simulink model "PID_sin_boques"  (Simulink 7.8)
settings: Solver=ode45  StartTime=0.0  StopTime=10  RelTol=1e-3
values from neighbouring files (symbols this model uses):
  b = 1.2*10^(-4)    (= 0.00012)    [Initial_datab.m]
  d = 3*10^(-6)    (= 3e-06)    [Initial_datab.m]
  Ixx = 10.4*10^(-3)    (= 0.0104)    [Initial_datab.m]
  Iyy = 11.2*10^(-3)    (= 0.0112)    [Initial_datab.m]
  Izz = 2.29*10^(-2)    (= 0.0229)    [Initial_datab.m]
  Jr = 7.25*10^(-5)    (= 7.25e-05)    [Initial_datab.m]
  Kp_phi = 4    [Const_PID.m]
  Kp_psi = 1.5    [Const_PID.m]
  Kp_theta = 2    [Const_PID.m]
  Kp_z = 8    [Const_PID.m]
  l = 0.225    [Initial_datab.m]
  m = 1.14    [Initial_datab.m]
  phi0 = 0    [Initial_datab.m]
  phi0dot = 0    [Initial_datab.m]
  psi0 = 0    [Initial_datab.m]
  psi0dot = 0    [Initial_datab.m]
  Td_phi = 0.1833    [Const_PID.m]
  Td_psi = 0.42    [Const_PID.m]
  Td_theta = 0.275    [Const_PID.m]
  Td_z = 0.5    [Const_PID.m]
  theta0 = 0    [Initial_datab.m]
  theta0dot = 0    [Initial_datab.m]
  Ti_phi = 100000000    [Const_PID.m]
  Ti_psi = 1000000    [Const_PID.m]
  Ti_theta = 10000000    [Const_PID.m]
  Ti_z = 1000000000    [Const_PID.m]
  x0 = 0    [Initial_datab.m]
  x0dot = 0    [Initial_datab.m]
  y0 = 0    [Initial_datab.m]
  y0dot = 0    [Initial_datab.m]
  z0 = 0    [Initial_datab.m]
  z0dot = 0    [Initial_datab.m]
undefined symbols (not defined in the file or in its folder): sigbuilder_block
libraries: aerolibconvert2 x9, simulink x1
settings Model: Creator=Ana  LastModifiedBy=Ana

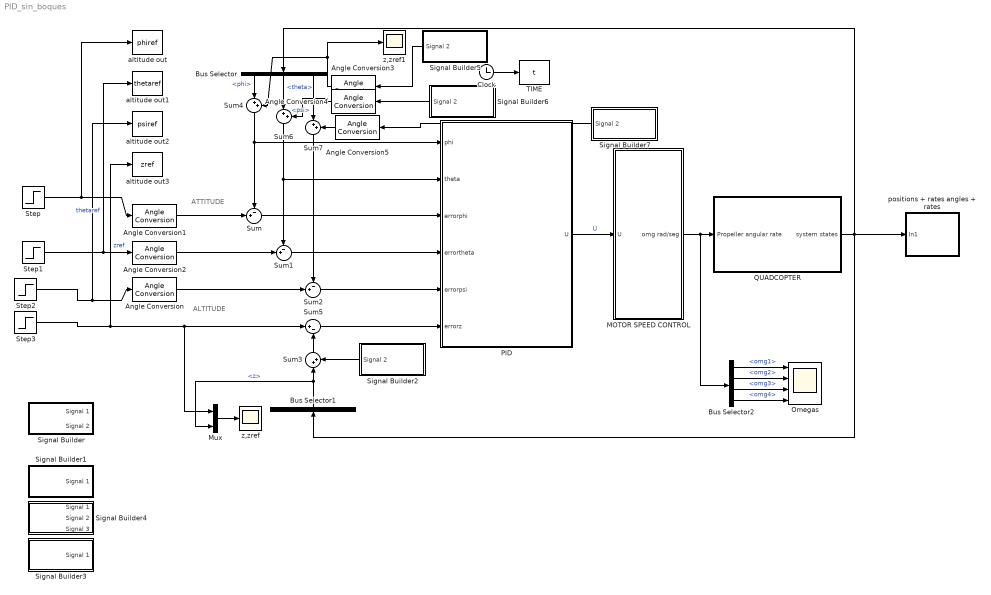
== system PID_sin_boques ==
  note: ATTITUDE
  note: ALTITUDE
  Angle Conversion{,1..5} (6 alike) : aerolibconvert2/Angle Conversion  IU=deg  OU=rad
  Bus Selector : BusSelector  OutputSignals=States.phi,States.theta,States.psi
  Bus Selector1 : BusSelector  OutputSignals=States.z
  Bus Selector2 : BusSelector  OutputSignals=omg1,omg2,omg3,omg4
  Clock : Clock
  MOTOR SPEED CONTROL : Subsystem
  Mux : Mux  Inputs=2
  Omegas : Scope  NumInputPorts=4
      settings: YMin=-5~-5~-5~-5  YMax=5~5~5~5  SaveName=ScopeData17
  PID : Subsystem
  QUADCOPTER : Subsystem
  Signal Builder : Subsystem  Tag=STV Subsys  LoadFcn=sigbuilder_block('load');  StartFcn=sigbuilder_block('start');  StopFcn=sigbuilder_block('stop');  ClipboardFcn=sigbuilder_block('clipboard');  mask(Sigbuilder block){}
      mask help: Simulink:masks:SigbuilderBlock_MD
      mask init:
      | if ~strcmp(get_param(bdroot(gcbh),'SimulationStatus'),'stopped') tuvar = sigbuilder_block('maskInit'); end
      settings: CopyFcn=sigbuilder_block('copy');  DeleteFcn=sigbuilder_block('delete');  ModelCloseFcn=sigbuilder_block('modelClose');  PreSaveFcn=sigbuilder_block('preSave');  NameChangeFcn=sigbuilder_block('namechange');  OpenFcn=sigbuilder_block('open',[437.25 117.75 550.5 394.5 ]);  CloseFcn=sigbuilder_block('close');
      mask Display: plot(0, 0, 100, 100,[2, 2, 32, 32, 2], [68, 8, 8, 68, 68],[32, 2], [38, 38], [32, 19, 2],[53, 60, 44], [32, 17, 17, 2],[16, 16, 31, 31]);txt = getActiveGroup(gcbh);text(2, 100, txt,'verticalAlignment', 'top');
  Signal Builder1 : Subsystem  Tag=STV Subsys  LoadFcn=sigbuilder_block('load');  StartFcn=sigbuilder_block('start');  StopFcn=sigbuilder_block('stop');  ClipboardFcn=sigbuilder_block('clipboard');  mask(Sigbuilder block){}
      mask help: Simulink:masks:SigbuilderBlock_MD
      mask init:
      | if ~strcmp(get_param(bdroot(gcbh),'SimulationStatus'),'stopped') tuvar = sigbuilder_block('maskInit'); end
      settings: CopyFcn=sigbuilder_block('copy');  DeleteFcn=sigbuilder_block('delete');  ModelCloseFcn=sigbuilder_block('modelClose');  PreSaveFcn=sigbuilder_block('preSave');  NameChangeFcn=sigbuilder_block('namechange');  OpenFcn=sigbuilder_block('open',[437.25 117.75 550.5 394.5 ]);  CloseFcn=sigbuilder_block('close');
      mask Display: plot(0, 0, 100, 100,[2, 2, 32, 32, 2], [68, 8, 8, 68, 68],[32, 2], [38, 38], [32, 19, 2],[53, 60, 44], [32, 17, 17, 2],[16, 16, 31, 31]);txt = getActiveGroup(gcbh);text(2, 100, txt,'verticalAlignment', 'top');
  Signal Builder2 : Subsystem  Tag=STV Subsys  LoadFcn=sigbuilder_block('load');  StartFcn=sigbuilder_block('start');  StopFcn=sigbuilder_block('stop');  ClipboardFcn=sigbuilder_block('clipboard');  mask(Sigbuilder block){}
      mask help: Simulink:masks:SigbuilderBlock_MD
      mask init:
      | if ~strcmp(get_param(bdroot(gcbh),'SimulationStatus'),'stopped') tuvar = sigbuilder_block('maskInit'); end
      settings: CopyFcn=sigbuilder_block('copy');  DeleteFcn=sigbuilder_block('delete');  ModelCloseFcn=sigbuilder_block('modelClose');  PreSaveFcn=sigbuilder_block('preSave');  NameChangeFcn=sigbuilder_block('namechange');  OpenFcn=sigbuilder_block('open',[437.25 117.75 550.5 394.5 ]);  CloseFcn=sigbuilder_block('close');
      mask Display: plot(0, 0, 100, 100,[2, 2, 32, 32, 2], [68, 8, 8, 68, 68],[32, 2], [38, 38], [32, 19, 2],[53, 60, 44], [32, 17, 17, 2],[16, 16, 31, 31]);txt = getActiveGroup(gcbh);text(2, 100, txt,'verticalAlignment', 'top');
  Signal Builder3 : Subsystem  Tag=STV Subsys  LoadFcn=sigbuilder_block('load');  StartFcn=sigbuilder_block('start');  StopFcn=sigbuilder_block('stop');  ClipboardFcn=sigbuilder_block('clipboard');  mask(Sigbuilder block){}
      mask help: Simulink:masks:SigbuilderBlock_MD
      mask init:
      | if ~strcmp(get_param(bdroot(gcbh),'SimulationStatus'),'stopped') tuvar = sigbuilder_block('maskInit'); end
      settings: CopyFcn=sigbuilder_block('copy');  DeleteFcn=sigbuilder_block('delete');  ModelCloseFcn=sigbuilder_block('modelClose');  PreSaveFcn=sigbuilder_block('preSave');  NameChangeFcn=sigbuilder_block('namechange');  OpenFcn=sigbuilder_block('open',[437.25 117.75 550.5 394.5 ]);  CloseFcn=sigbuilder_block('close');
      mask Display: plot(0, 0, 100, 100,[2, 2, 32, 32, 2], [68, 8, 8, 68, 68],[32, 2], [38, 38], [32, 19, 2],[53, 60, 44], [32, 17, 17, 2],[16, 16, 31, 31]);txt = getActiveGroup(gcbh);text(2, 100, txt,'verticalAlignment', 'top');
  Signal Builder4 : Subsystem  Tag=STV Subsys  LoadFcn=sigbuilder_block('load');  StartFcn=sigbuilder_block('start');  StopFcn=sigbuilder_block('stop');  ClipboardFcn=sigbuilder_block('clipboard');  mask(Sigbuilder block){}
      mask help: Simulink:masks:SigbuilderBlock_MD
      mask init:
      | if ~strcmp(get_param(bdroot(gcbh),'SimulationStatus'),'stopped') tuvar = sigbuilder_block('maskInit'); end
      settings: CopyFcn=sigbuilder_block('copy');  DeleteFcn=sigbuilder_block('delete');  ModelCloseFcn=sigbuilder_block('modelClose');  PreSaveFcn=sigbuilder_block('preSave');  NameChangeFcn=sigbuilder_block('namechange');  OpenFcn=sigbuilder_block('open',[437.25 117.75 550.5 394.5 ]);  CloseFcn=sigbuilder_block('close');
      mask Display: plot(0, 0, 100, 100,[2, 2, 32, 32, 2], [68, 8, 8, 68, 68],[32, 2], [38, 38], [32, 19, 2],[53, 60, 44], [32, 17, 17, 2],[16, 16, 31, 31]);txt = getActiveGroup(gcbh);text(2, 100, txt,'verticalAlignment', 'top');
  Signal Builder5 : Subsystem  Tag=STV Subsys  LoadFcn=sigbuilder_block('load');  StartFcn=sigbuilder_block('start');  StopFcn=sigbuilder_block('stop');  ClipboardFcn=sigbuilder_block('clipboard');  mask(Sigbuilder block){}
      mask help: Simulink:masks:SigbuilderBlock_MD
      mask init:
      | if ~strcmp(get_param(bdroot(gcbh),'SimulationStatus'),'stopped') tuvar = sigbuilder_block('maskInit'); end
      settings: CopyFcn=sigbuilder_block('copy');  DeleteFcn=sigbuilder_block('delete');  ModelCloseFcn=sigbuilder_block('modelClose');  PreSaveFcn=sigbuilder_block('preSave');  NameChangeFcn=sigbuilder_block('namechange');  OpenFcn=sigbuilder_block('open',[437.25 117.75 550.5 394.5 ]);  CloseFcn=sigbuilder_block('close');
      mask Display: plot(0, 0, 100, 100,[2, 2, 32, 32, 2], [68, 8, 8, 68, 68],[32, 2], [38, 38], [32, 19, 2],[53, 60, 44], [32, 17, 17, 2],[16, 16, 31, 31]);txt = getActiveGroup(gcbh);text(2, 100, txt,'verticalAlignment', 'top');
  Signal Builder6 : Subsystem  Tag=STV Subsys  LoadFcn=sigbuilder_block('load');  StartFcn=sigbuilder_block('start');  StopFcn=sigbuilder_block('stop');  ClipboardFcn=sigbuilder_block('clipboard');  mask(Sigbuilder block){}
      mask help: Simulink:masks:SigbuilderBlock_MD
      mask init:
      | if ~strcmp(get_param(bdroot(gcbh),'SimulationStatus'),'stopped') tuvar = sigbuilder_block('maskInit'); end
      settings: CopyFcn=sigbuilder_block('copy');  DeleteFcn=sigbuilder_block('delete');  ModelCloseFcn=sigbuilder_block('modelClose');  PreSaveFcn=sigbuilder_block('preSave');  NameChangeFcn=sigbuilder_block('namechange');  OpenFcn=sigbuilder_block('open',[437.25 117.75 550.5 394.5 ]);  CloseFcn=sigbuilder_block('close');
      mask Display: plot(0, 0, 100, 100,[2, 2, 32, 32, 2], [68, 8, 8, 68, 68],[32, 2], [38, 38], [32, 19, 2],[53, 60, 44], [32, 17, 17, 2],[16, 16, 31, 31]);txt = getActiveGroup(gcbh);text(2, 100, txt,'verticalAlignment', 'top');
  Signal Builder7 : Subsystem  Tag=STV Subsys  LoadFcn=sigbuilder_block('load');  StartFcn=sigbuilder_block('start');  StopFcn=sigbuilder_block('stop');  ClipboardFcn=sigbuilder_block('clipboard');  mask(Sigbuilder block){}
      mask help: Simulink:masks:SigbuilderBlock_MD
      mask init:
      | if ~strcmp(get_param(bdroot(gcbh),'SimulationStatus'),'stopped') tuvar = sigbuilder_block('maskInit'); end
      settings: CopyFcn=sigbuilder_block('copy');  DeleteFcn=sigbuilder_block('delete');  ModelCloseFcn=sigbuilder_block('modelClose');  PreSaveFcn=sigbuilder_block('preSave');  NameChangeFcn=sigbuilder_block('namechange');  OpenFcn=sigbuilder_block('open',[437.25 117.75 550.5 394.5 ]);  CloseFcn=sigbuilder_block('close');
      mask Display: plot(0, 0, 100, 100,[2, 2, 32, 32, 2], [68, 8, 8, 68, 68],[32, 2], [38, 38], [32, 19, 2],[53, 60, 44], [32, 17, 17, 2],[16, 16, 31, 31]);txt = getActiveGroup(gcbh);text(2, 100, txt,'verticalAlignment', 'top');
  Step{,1..3} (4 alike) : Step  SampleTime=0
  Sum : Sum  Inputs=-+|
  Sum1 : Sum  Inputs=-+|
  Sum2 : Sum  Inputs=-+|
  Sum{3..4,6..7} (4 alike) : Sum  Inputs=|++
  Sum5 : Sum  Inputs=|+-
  TIME : ToWorkspace  VariableName=t  SampleTime=-1  SaveFormat=Array
  altitude out : ToWorkspace  VariableName=phiref  SampleTime=-1  SaveFormat=Array
  altitude out1 : ToWorkspace  VariableName=thetaref  SampleTime=-1  SaveFormat=Array
  altitude out2 : ToWorkspace  VariableName=psiref  SampleTime=-1  SaveFormat=Array
  altitude out3 : ToWorkspace  VariableName=zref  SampleTime=-1  SaveFormat=Array
  positions + rates angles + rates : Subsystem
      mask Display: disp('system states')
  z,zref : Scope
      settings: YMin=8.5  YMax=17.5  SaveName=ScopeData3
  z,zref1 : Scope
      settings: YMin=8.5  YMax=17.5  SaveName=ScopeData18
  wires:
  QUADCOPTER/1(system states) -> Bus Selector/1, Bus Selector1/1, positions + rates angles + rates/1(In1)
  Bus Selector/1 -> Sum4/1  "<phi>"
  Step1/1 -> Angle Conversion2/1, altitude out1/1  "thetaref"
  Sum/1 -> PID/3(errorphi)
  Sum1/1 -> PID/4(errortheta)
  Sum2/1 -> PID/5(errorpsi)
  PID/1(U) -> MOTOR SPEED CONTROL/1(U)  "U"
  Step3/1 -> Sum5/1, Mux/1, altitude out3/1  "zref"
  Mux/1 -> z,zref/1
  Sum5/1 -> PID/6(errorz)
  Angle Conversion/1 -> Sum2/2
  Angle Conversion2/1 -> Sum1/2
  Angle Conversion1/1 -> Sum/2
  Bus Selector1/1 -> Sum3/1, Mux/2  "<z>"
  Sum3/1 -> Sum5/2
  Sum4/1 -> Sum/1, PID/1(phi)
  Bus Selector/2 -> Sum6/1  "<theta>"
  Sum6/1 -> Sum1/1, PID/2(theta)
  Bus Selector/3 -> Sum7/1  "<psi>"
  Sum7/1 -> Sum2/1
  Clock/1 -> TIME/1
  MOTOR SPEED CONTROL/1(omg rad/seg) -> QUADCOPTER/1(Propeller angular rate), Bus Selector2/1
  Bus Selector2/1 -> Omegas/1  "<omg1>"
  Bus Selector2/2 -> Omegas/2  "<omg2>"
  Bus Selector2/3 -> Omegas/3  "<omg3>"
  Bus Selector2/4 -> Omegas/4  "<omg4>"
  Step2/1 -> Angle Conversion/1, altitude out2/1
  Step/1 -> Angle Conversion1/1, altitude out/1
  Signal Builder6/1(Signal 2) -> Angle Conversion4/1
  Signal Builder7/1(Signal 2) -> Angle Conversion5/1
  Angle Conversion3/1 -> z,zref1/1, Sum4/2
  Angle Conversion5/1 -> Sum7/2
  Angle Conversion4/1 -> Sum6/2
  Signal Builder2/1(Signal 2) -> Sum3/2
  Signal Builder5/1(Signal 2) -> Angle Conversion3/1

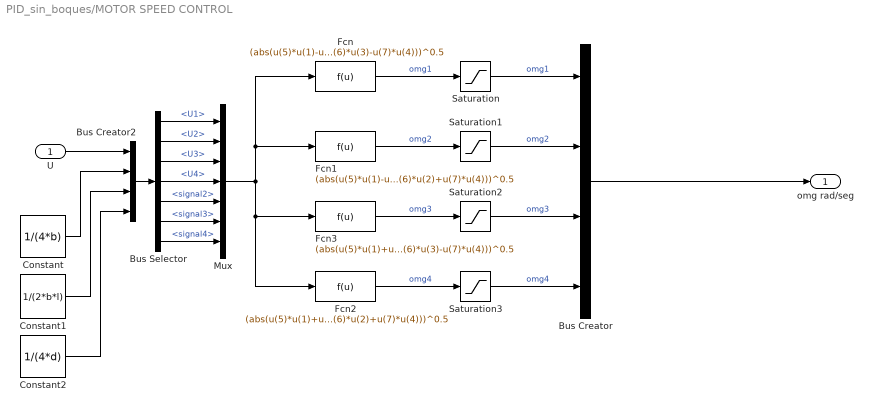
== system PID_sin_boques/MOTOR SPEED CONTROL ==
  U : Inport
  Bus Creator : BusCreator
  Bus Creator2 : BusCreator
  Bus Selector : BusSelector  OutputSignals=U.U1,U.U2,U.U3,U.U4,signal2,signal3,signal4
  Constant : Constant  Value=1/(4*b)
  Constant1 : Constant  Value=1/(2*b*l)
  Constant2 : Constant  Value=1/(4*d)
  Fcn : Fcn  Expr=(abs(u(5)*u(1)-u(6)*u(3)-u(7)*u(4)))^0.5
  Fcn1 : Fcn  Expr=(abs(u(5)*u(1)-u(6)*u(2)+u(7)*u(4)))^0.5
  Fcn2 : Fcn  Expr=(abs(u(5)*u(1)+u(6)*u(2)+u(7)*u(4)))^0.5
  Fcn3 : Fcn  Expr=(abs(u(5)*u(1)+u(6)*u(3)-u(7)*u(4)))^0.5
  Mux : Mux  Inputs=7
  Saturation{,1..3} (4 alike) : Saturate  UpperLimit=215.86  LowerLimit=0  ZeroCross=off
  omg rad/seg : Outport
  wires:
  Constant/1 -> Bus Creator2/2
  Constant1/1 -> Bus Creator2/3
  Bus Creator2/1 -> Bus Selector/1
  Constant2/1 -> Bus Creator2/4
  Bus Selector/1 -> Mux/1  "<U1>"
  Bus Selector/2 -> Mux/2  "<U2>"
  Bus Selector/3 -> Mux/3  "<U3>"
  Bus Selector/4 -> Mux/4  "<U4>"
  Bus Selector/5 -> Mux/5  "<signal2>"
  Bus Selector/6 -> Mux/6  "<signal3>"
  Bus Selector/7 -> Mux/7  "<signal4>"
  U/1 -> Bus Creator2/1
  Bus Creator/1 -> omg rad/seg/1
  Fcn/1 -> Saturation/1  "omg1"
  Fcn1/1 -> Saturation1/1  "omg2"
  Fcn3/1 -> Saturation2/1  "omg3"
  Fcn2/1 -> Saturation3/1  "omg4"
  Saturation/1 -> Bus Creator/1  "omg1"
  Saturation1/1 -> Bus Creator/2  "omg2"
  Saturation2/1 -> Bus Creator/3  "omg3"
  Saturation3/1 -> Bus Creator/4  "omg4"
  Mux/1 -> Fcn1/1, Fcn/1, Fcn3/1, Fcn2/1

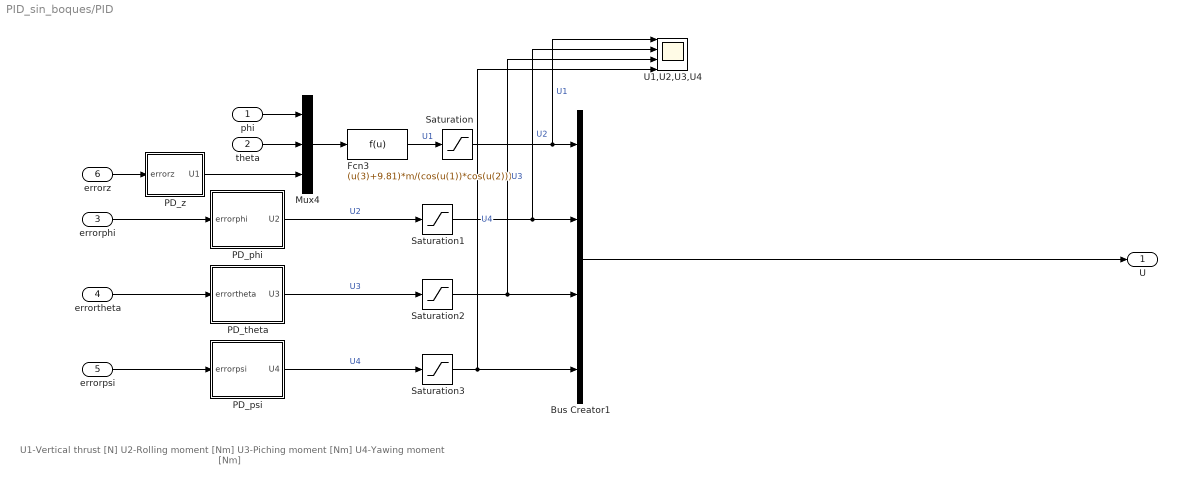
== system PID_sin_boques/PID ==
  note: U1-Vertical thrust [N]
      | U2-Rolling moment [Nm]
      | U3-Piching moment [Nm]
      | U4-Yawing moment [Nm]
  phi : Inport
  theta : Inport  Port=2
  errorphi : Inport  Port=3
  errortheta : Inport  Port=4
  errorpsi : Inport  Port=5
  errorz : Inport  Port=6
  Bus Creator1 : BusCreator
  Fcn3 : Fcn  Expr=(u(3)+9.81)*m/(cos(u(1))*cos(u(2)))
  Mux4 : Mux  Inputs=3
  PD_phi : Subsystem
  PD_psi : Subsystem
  PD_theta : Subsystem
  PD_z : Subsystem
  Saturation : Saturate  UpperLimit=22.36  LowerLimit=0  ZeroCross=off
  Saturation1 : Saturate  UpperLimit=5.5915  LowerLimit=-5.5915  ZeroCross=off
  Saturation2 : Saturate  UpperLimit=5.5915  LowerLimit=-5.5915  ZeroCross=off
  Saturation3 : Saturate  UpperLimit=5.5915  LowerLimit=-5.5915  ZeroCross=off
  U1,U2,U3,U4 : Scope  NumInputPorts=4
      settings: YMin=-5~-5~-5~-5  YMax=5~5~5~5  SaveName=ScopeData22
  U : Outport
  wires:
  Bus Creator1/1 -> U/1
  errorphi/1 -> PD_phi/1(errorphi)
  errortheta/1 -> PD_theta/1(errortheta)
  errorpsi/1 -> PD_psi/1(errorpsi)
  PD_psi/1(U4) -> Saturation3/1  "U4"
  PD_theta/1(U3) -> Saturation2/1  "U3"
  PD_phi/1(U2) -> Saturation1/1  "U2"
  Fcn3/1 -> Saturation/1  "U1"
  Mux4/1 -> Fcn3/1
  errorz/1 -> PD_z/1(errorz)
  PD_z/1(U1) -> Mux4/3
  theta/1 -> Mux4/2
  phi/1 -> Mux4/1
  Saturation/1 -> Bus Creator1/1, U1,U2,U3,U4/1  "U1"
  Saturation1/1 -> Bus Creator1/2, U1,U2,U3,U4/2  "U2"
  Saturation2/1 -> Bus Creator1/3, U1,U2,U3,U4/3  "U3"
  Saturation3/1 -> Bus Creator1/4, U1,U2,U3,U4/4  "U4"

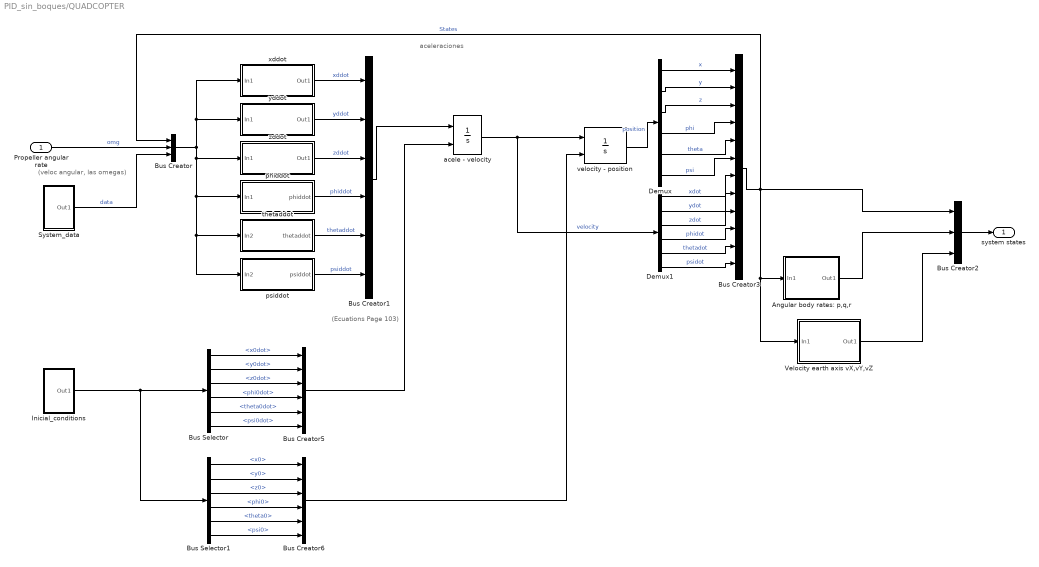
== system PID_sin_boques/QUADCOPTER ==
  note: aceleraciones
  note: (Ecuations Page 103)
  note: (veloc angular, las omegas)
  Propeller angular rate : Inport
  Angular body rates: p,q,r : Subsystem
  Bus Creator : BusCreator  Inputs=3
  Bus Creator1 : BusCreator  Inputs=6
  Bus Creator2 : BusCreator  Inputs=3
  Bus Creator3 : BusCreator  Inputs=12
  Bus Creator5 : BusCreator  Inputs=6
  Bus Creator6 : BusCreator  Inputs=6
  Bus Selector : BusSelector  OutputSignals=x0dot,y0dot,z0dot,phi0dot,theta0dot,psi0dot
  Bus Selector1 : BusSelector  OutputSignals=x0,y0,z0,phi0,theta0,psi0
  Demux : Demux  Outputs=6
  Demux1 : Demux  Outputs=6
  Inicial_conditions : Subsystem
  System_data : Subsystem
  Velocity earth axis vX,vY,vZ : Subsystem
  acele - velocity : Integrator  InitialConditionSource=external
  phiddot : Subsystem
  psiddot : Subsystem
  thetaddot : Subsystem
  velocity - position : Integrator  InitialConditionSource=external
  xddot : Subsystem
  yddot : Subsystem
  zddot : Subsystem
  system states : Outport
  wires:
  Demux/1 -> Bus Creator3/1  "x"
  Demux/2 -> Bus Creator3/2  "y"
  Demux/3 -> Bus Creator3/3  "z"
  Demux1/1 -> Bus Creator3/7  "xdot"
  Demux1/2 -> Bus Creator3/8  "ydot"
  Demux1/3 -> Bus Creator3/9  "zdot"
  Demux1/4 -> Bus Creator3/10  "phidot"
  Demux1/5 -> Bus Creator3/11  "thetadot"
  Demux1/6 -> Bus Creator3/12  "psidot"
  Bus Creator3/1 -> Bus Creator/1, Bus Creator2/1, Angular body rates: p,q,r/1(In1), Velocity earth axis vX,vY,vZ/1(In1)  "States"
  Bus Selector/1 -> Bus Creator5/1  "<x0dot>"
  Bus Selector/2 -> Bus Creator5/2  "<y0dot>"
  Bus Selector/3 -> Bus Creator5/3  "<z0dot>"
  Bus Selector/4 -> Bus Creator5/4  "<phi0dot>"
  Bus Selector/5 -> Bus Creator5/5  "<theta0dot>"
  Bus Selector/6 -> Bus Creator5/6  "<psi0dot>"
  Bus Selector1/1 -> Bus Creator6/1  "<x0>"
  Bus Selector1/2 -> Bus Creator6/2  "<y0>"
  Bus Selector1/3 -> Bus Creator6/3  "<z0>"
  Bus Selector1/4 -> Bus Creator6/4  "<phi0>"
  Bus Selector1/5 -> Bus Creator6/5  "<theta0>"
  Bus Selector1/6 -> Bus Creator6/6  "<psi0>"
  Bus Creator5/1 -> acele - velocity/2
  velocity - position/1 -> Demux/1  "position"
  Bus Creator6/1 -> velocity - position/2
  acele - velocity/1 -> velocity - position/1, Demux1/1  "velocity"
  yddot/1(Out1) -> Bus Creator1/2  "yddot"
  zddot/1(Out1) -> Bus Creator1/3  "zddot"
  phiddot/1(phiddot) -> Bus Creator1/4  "phiddot"
  thetaddot/1(thetaddot) -> Bus Creator1/5  "thetaddot"
  psiddot/1(psiddot) -> Bus Creator1/6  "psiddot"
  Bus Creator1/1 -> acele - velocity/1
  xddot/1(Out1) -> Bus Creator1/1  "xddot"
  Propeller angular rate/1 -> Bus Creator/2  "omg"
  System_data/1(Out1) -> Bus Creator/3  "data"
  Bus Creator/1 -> xddot/1(In1), yddot/1(In1), thetaddot/1(In2), psiddot/1(In2), phiddot/1(In1), zddot/1(In1)
  Angular body rates: p,q,r/1(Out1) -> Bus Creator2/2
  Bus Creator2/1 -> system states/1
  Inicial_conditions/1(Out1) -> Bus Selector/1, Bus Selector1/1
  Velocity earth axis vX,vY,vZ/1(Out1) -> Bus Creator2/3
  Demux/4 -> Bus Creator3/4  "phi"
  Demux/6 -> Bus Creator3/6  "psi"
  Demux/5 -> Bus Creator3/5  "theta"

== system PID_sin_boques/Signal Builder ==
  Demux : Demux  Tag=STV Demux  Outputs=2
  FromWs : FromWorkspace  Tag=STV FromWs  VariableName=tuvar  SampleTime=0  SigBuilderData=DataTag0  VnvData=DataTag1
      SigBuilderData=|
      | common.afterFinalStr = 'Extrapolate'
      | common.sampleTime = 0
      | dataSet.timeRange = [0 10]
      | dataSet.name = 'Group 1'
      | sbobj.Groups.Name = 'Group 1'
      | sbobj.Groups.Signals(1).Name = 'Signal 1'
      | sbobj.Groups.Signals(1).XData = [0 2 4 6 8 10]
      | sbobj.Groups.Signals(1).YData = [0 0 1 1 0 0]
      | sbobj.Groups.Signals(2).Name = 'Signal 2'
      | sbobj.Groups.Signals(2).XData = [0 0.5 1 1.5 2 2.5 3 3.5 4 4.5 5 5.5 6 6.5 7 7.5 8 8.5 9 9.5 10]
      | sbobj.Groups.Signals(2).YData = [0 0.707106781187 1 0.707106781187 1.22464679915e-16 -0.707106781187 -1 -0.707106781187 0 0.707106781187 1 0.707106781187 1.22464679915e-16 -0.707106781187 -1 -0.707106781187 0 0.707106781187 1 0.707106781187 1.22464679915e-16]
  Signal 1 : Outport  Tag=STV Outport
  Signal 2 : Outport  Tag=STV Outport  Port=2
  wires:
  Demux/1 -> Signal 1/1
  FromWs/1 -> Demux/1
  Demux/2 -> Signal 2/1

== system PID_sin_boques/Signal Builder1 ==
  Demux : Demux  Tag=STV Demux  Outputs=1
  FromWs : FromWorkspace  Tag=STV FromWs  VariableName=tuvar  SampleTime=0  SigBuilderData=DataTag2  VnvData=DataTag3
      SigBuilderData=|
      | common.afterFinalStr = 'Extrapolate'
      | common.sampleTime = 0
      | dataSet.timeRange = [0 10]
      | dataSet.name = 'Group 1'
      | sbobj.Groups.Name = 'Group 1'
      | sbobj.Groups.Signals.Name = 'Signal 1'
      | sbobj.Groups.Signals.XData = [0 4 6 6 10]
      | sbobj.Groups.Signals.YData = [0 1 1 0.5 0]
  Signal 1 : Outport  Tag=STV Outport
  wires:
  Demux/1 -> Signal 1/1
  FromWs/1 -> Demux/1

== system PID_sin_boques/Signal Builder2 ==
  Demux : Demux  Tag=STV Demux  Outputs=1
  FromWs : FromWorkspace  Tag=STV FromWs  VariableName=tuvar  SampleTime=0  SigBuilderData=DataTag4  VnvData=DataTag5
      SigBuilderData=|
      | common.afterFinalStr = 'Extrapolate'
      | common.sampleTime = 0
      | dataSet.timeRange = [0 10]
      | dataSet.name = 'Group 1'
      | sbobj.Groups.Name = 'Group 1'
      | sbobj.Groups.Signals.Name = 'Signal 2'
      | sbobj.Groups.Signals.XData = [0 3 3 3.5 3.5 10]
      | sbobj.Groups.Signals.YData = [0 0 1 1 0 0]
  Signal 2 : Outport  Tag=STV Outport
  wires:
  FromWs/1 -> Demux/1
  Demux/1 -> Signal 2/1

== system PID_sin_boques/Signal Builder3 ==
  Demux : Demux  Tag=STV Demux  Outputs=1
  FromWs : FromWorkspace  Tag=STV FromWs  VariableName=tuvar  SampleTime=0  SigBuilderData=DataTag6  VnvData=DataTag7
      SigBuilderData=|
      | common.afterFinalStr = 'Extrapolate'
      | common.sampleTime = 0
      | dataSet.timeRange = [0 10]
      | dataSet.name = 'Group 1'
      | sbobj.Groups.Name = 'Group 1'
      | sbobj.Groups.Signals.Name = 'Signal 1'
      | sbobj.Groups.Signals.XData = [0 3 4 6 8 10]
      | sbobj.Groups.Signals.YData = [0 1 1.98 1.98 0.5 0]
  Signal 1 : Outport  Tag=STV Outport
  wires:
  Demux/1 -> Signal 1/1
  FromWs/1 -> Demux/1

== system PID_sin_boques/Signal Builder4 ==
  Demux : Demux  Tag=STV Demux  Outputs=3
  FromWs : FromWorkspace  Tag=STV FromWs  VariableName=tuvar  SampleTime=0  SigBuilderData=DataTag8  VnvData=DataTag9
      SigBuilderData=|
      | common.afterFinalStr = 'Extrapolate'
      | common.sampleTime = 0
      | dataSet.timeRange = [0 10]
      | dataSet.name = 'Group 1'
      | sbobj.Groups.Name = 'Group 1'
      | sbobj.Groups.Signals(1).Name = 'Signal 1'
      | sbobj.Groups.Signals(1).XData = [0 2 4 6 8 10]
      | sbobj.Groups.Signals(1).YData = [0 0 1 1 0 0]
      | sbobj.Groups.Signals(2).Name = 'Signal 2'
      | sbobj.Groups.Signals(2).XData = [0 4 4 6 6 10]
      | sbobj.Groups.Signals(2).YData = [0 0 1 1 0 0]
      | sbobj.Groups.Signals(3).Name = 'Signal 3'
      | sbobj.Groups.Signals(3).XData = [0 1 2 2 4 4 6 6 8 8 8.56 10]
      | sbobj.Groups.Signals(3).YData = [0 0 0 1 1 0 0 1 1 0 0 0]
  Signal 1 : Outport  Tag=STV Outport
  Signal 2 : Outport  Tag=STV Outport  Port=2
  Signal 3 : Outport  Tag=STV Outport  Port=3
  wires:
  FromWs/1 -> Demux/1
  Demux/1 -> Signal 1/1
  Demux/2 -> Signal 2/1
  Demux/3 -> Signal 3/1

== system PID_sin_boques/Signal Builder5 ==
  Demux : Demux  Tag=STV Demux  Outputs=1
  FromWs : FromWorkspace  Tag=STV FromWs  VariableName=tuvar  SampleTime=0  SigBuilderData=DataTag10  VnvData=DataTag11
      SigBuilderData=|
      | common.afterFinalStr = 'Extrapolate'
      | common.sampleTime = 0
      | dataSet.timeRange = [0 10]
      | dataSet.name = 'Group 1'
      | sbobj.Groups.Name = 'Group 1'
      | sbobj.Groups.Signals.Name = 'Signal 2'
      | sbobj.Groups.Signals.XData = [0 5 5 5.5 5.5 10]
      | sbobj.Groups.Signals.YData = [0 0 3 3 0 0]
  Signal 2 : Outport  Tag=STV Outport
  wires:
  FromWs/1 -> Demux/1
  Demux/1 -> Signal 2/1

== system PID_sin_boques/Signal Builder6 ==
  Demux : Demux  Tag=STV Demux  Outputs=1
  FromWs : FromWorkspace  Tag=STV FromWs  VariableName=tuvar  SampleTime=0  SigBuilderData=DataTag12  VnvData=DataTag13
      SigBuilderData=|
      | common.afterFinalStr = 'Extrapolate'
      | common.sampleTime = 0
      | dataSet.timeRange = [0 10]
      | dataSet.name = 'Group 1'
      | sbobj.Groups.Name = 'Group 1'
      | sbobj.Groups.Signals.Name = 'Signal 2'
      | sbobj.Groups.Signals.XData = [0 7 7 7.5 7.5 10]
      | sbobj.Groups.Signals.YData = [0 0 3 3 0 0]
  Signal 2 : Outport  Tag=STV Outport
  wires:
  FromWs/1 -> Demux/1
  Demux/1 -> Signal 2/1

== system PID_sin_boques/Signal Builder7 ==
  Demux : Demux  Tag=STV Demux  Outputs=1
  FromWs : FromWorkspace  Tag=STV FromWs  VariableName=tuvar  SampleTime=0  SigBuilderData=DataTag14  VnvData=DataTag15
      SigBuilderData=|
      | common.afterFinalStr = 'Extrapolate'
      | common.sampleTime = 0
      | dataSet.timeRange = [0 10]
      | dataSet.name = 'Group 1'
      | sbobj.Groups.Name = 'Group 1'
      | sbobj.Groups.Signals.Name = 'Signal 2'
      | sbobj.Groups.Signals.XData = [0 9 9 9.5 9.5 10]
      | sbobj.Groups.Signals.YData = [0 0 3 3 0 0]
  Signal 2 : Outport  Tag=STV Outport
  wires:
  FromWs/1 -> Demux/1
  Demux/1 -> Signal 2/1

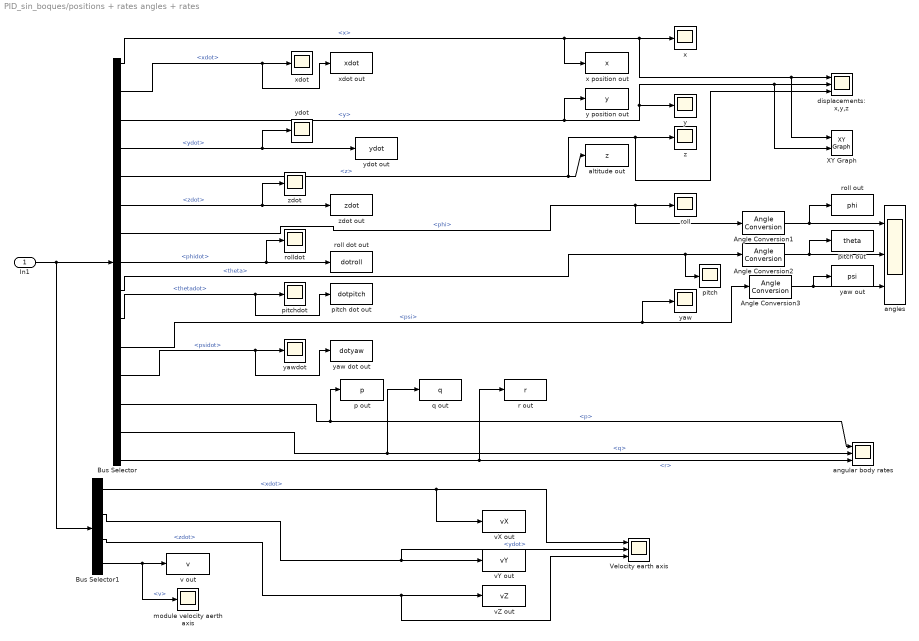
== system PID_sin_boques/positions + rates angles + rates ==
  In1 : Inport
  Angle Conversion1 : aerolibconvert2/Angle Conversion  IU=rad  OU=deg
  Angle Conversion2 : aerolibconvert2/Angle Conversion  IU=rad  OU=deg
  Angle Conversion3 : aerolibconvert2/Angle Conversion  IU=rad  OU=deg
  Bus Selector : BusSelector  OutputSignals=States.x,States.xdot,States.y,States.ydot,States.z,States.zdot,States.phi,States.phidot,States.theta,States.thetadot,States.psi,States.psidot,signal2.p,signal2.q,signal2.r
  Bus Selector1 : BusSelector  OutputSignals=States.xdot,States.ydot,States.zdot,signal3.v
  Velocity earth axis : Scope  NumInputPorts=3
      settings: TimeRange=0.5  YMin=-2.92169e+092~-1.59453e+092~5.72254e+092  YMax=-2.64343e+092~-1.44267e+092~6.32492e+092  SaveName=ScopeData15
  XY Graph : simulink/Sinks/XY Graph  xmin=-8  xmax=8  ymin=-8  ymax=8  st=-1
  altitude out : ToWorkspace  VariableName=z  SampleTime=-1  SaveFormat=Array
  angles : Scope  NumInputPorts=3
      settings: TimeRange=0.1  YMin=0.951985~0.949043~0.952413  YMax=1.05219~1.04894~1.05267  SaveName=ScopeData13
  angular body rates : Scope  NumInputPorts=3
      settings: TimeRange=5  YMin=-5~-0.02~-0.001  YMax=20~0.005000000000000001~0.004  SaveName=ScopeData14
  displacements: x,y,z : Scope  NumInputPorts=3
      settings: TimeRange=0.5  YMin=-1~-1~5.425  YMax=1~1~5.65  SaveName=ScopeData19
  module velocity aerth axis : Scope
      settings: SaveName=ScopeData16
  p out : ToWorkspace  VariableName=p  SampleTime=-1  SaveFormat=Structure
  pitch : Scope
      settings: TimeRange=4  YMin=-0.055  YMax=0.045
  pitch dot out : ToWorkspace  VariableName=dotpitch  SampleTime=-1  SaveFormat=Array
  pitch out : ToWorkspace  VariableName=theta  SampleTime=-1  SaveFormat=Array
  pitchdot : Scope
      settings: YMin=-1.75  YMax=1.75  SaveName=ScopeData4
  q out : ToWorkspace  VariableName=q  SampleTime=-1  SaveFormat=Structure
  r out : ToWorkspace  VariableName=r  SampleTime=-1  SaveFormat=Structure
  roll : Scope
      settings: TimeRange=0.25  YMin=-0.031  YMax=-0.008
  roll dot out : ToWorkspace  VariableName=dotroll  SampleTime=-1  SaveFormat=Array
  roll out : ToWorkspace  VariableName=phi  SampleTime=-1  SaveFormat=Array
  rolldot : Scope
      settings: TimeRange=7  YMin=-0.15  YMax=0.125  SaveName=ScopeData5
  v out : ToWorkspace  VariableName=v  SampleTime=-1  SaveFormat=Array
  vX out : ToWorkspace  VariableName=vX  SampleTime=-1  SaveFormat=Array
  vY out : ToWorkspace  VariableName=vY  SampleTime=-1  SaveFormat=Array
  vZ out : ToWorkspace  VariableName=vZ  SampleTime=-1  SaveFormat=Array
  x : Scope
      settings: TimeRange=20  YMin=-0.5  YMax=2.5  SaveName=ScopeData6
  x position out : ToWorkspace  VariableName=x  SampleTime=-1  SaveFormat=Array
  xdot : Scope
      settings: TimeRange=5  YMin=-4.75e-015  YMax=0  SaveName=ScopeData7
  xdot out : ToWorkspace  VariableName=xdot  SampleTime=-1  SaveFormat=Array
  y : Scope
      settings: TimeRange=5  YMin=1.825  YMax=2.075  SaveName=ScopeData8
  y position out : ToWorkspace  VariableName=y  SampleTime=-1  SaveFormat=Array
  yaw : Scope
      settings: TimeRange=5  YMin=-0.02  YMax=0.0125  SaveName=ScopeData2
  yaw dot out : ToWorkspace  VariableName=dotyaw  SampleTime=-1  SaveFormat=Array
  yaw out : ToWorkspace  VariableName=psi  SampleTime=-1  SaveFormat=Array
  yawdot : Scope
      settings: TimeRange=18  YMin=-0.275  YMax=0.15  SaveName=ScopeData9
  ydot : Scope
      settings: TimeRange=5  YMin=-143.75  YMax=-141.75  SaveName=ScopeData10
  ydot out : ToWorkspace  VariableName=ydot  SampleTime=-1  SaveFormat=Array
  z : Scope
      settings: TimeRange=5  YMin=0.2  YMax=1.5  SaveName=ScopeData11
  zdot : Scope
      settings: TimeRange=10  YMin=-110.5  YMax=-107.25  SaveName=ScopeData12
  zdot out : ToWorkspace  VariableName=zdot  SampleTime=-1  SaveFormat=Array
  wires:
  Bus Selector/3 -> y position out/1, y/1, displacements: x,y,z/2, XY Graph/2  "<y>"
  Bus Selector/12 -> yawdot/1, yaw dot out/1  "<psidot>"
  In1/1 -> Bus Selector/1, Bus Selector1/1
  Bus Selector/10 -> pitchdot/1, pitch dot out/1  "<thetadot>"
  Bus Selector/15 -> angular body rates/3, r out/1  "<r>"
  Bus Selector/14 -> angular body rates/2, q out/1  "<q>"
  Bus Selector/13 -> angular body rates/1, p out/1  "<p>"
  Bus Selector/1 -> x position out/1, x/1, displacements: x,y,z/1, XY Graph/1  "<x>"
  Bus Selector/2 -> xdot out/1, xdot/1  "<xdot>"
  Bus Selector/4 -> ydot out/1, ydot/1  "<ydot>"
  Bus Selector/5 -> altitude out/1, z/1, displacements: x,y,z/3  "<z>"
  Bus Selector/6 -> zdot/1, zdot out/1  "<zdot>"
  Bus Selector/8 -> rolldot/1, roll dot out/1  "<phidot>"
  Bus Selector/9 -> pitch/1, Angle Conversion2/1  "<theta>"
  Bus Selector/11 -> yaw/1, Angle Conversion3/1  "<psi>"
  Bus Selector/7 -> roll/1, Angle Conversion1/1  "<phi>"
  Bus Selector1/2 -> vY out/1, Velocity earth axis/2  "<ydot>"
  Bus Selector1/3 -> vZ out/1, Velocity earth axis/3  "<zdot>"
  Bus Selector1/4 -> v out/1, module velocity aerth axis/1  "<v>"
  Bus Selector1/1 -> vX out/1, Velocity earth axis/1  "<xdot>"
  Angle Conversion1/1 -> angles/1, roll out/1
  Angle Conversion2/1 -> angles/2, pitch out/1
  Angle Conversion3/1 -> angles/3, yaw out/1

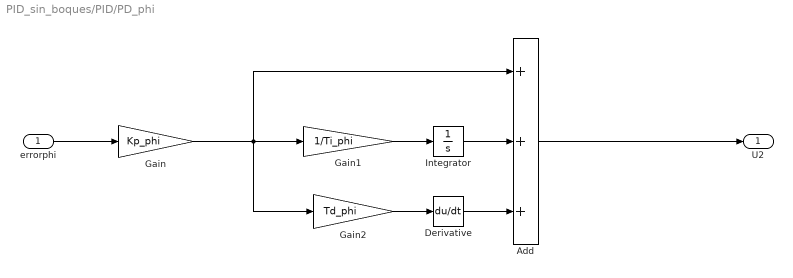
== system PID_sin_boques/PID/PD_phi ==
  errorphi : Inport
  Add : Sum  Inputs=+++
  Derivative : Derivative
  Gain : Gain  Gain=Kp_phi
  Gain1 : Gain  Gain=1/Ti_phi
  Gain2 : Gain  Gain=Td_phi
  Integrator : Integrator
  U2 : Outport
  wires:
  errorphi/1 -> Gain/1
  Add/1 -> U2/1
  Gain/1 -> Add/1, Gain1/1, Gain2/1
  Gain1/1 -> Integrator/1
  Integrator/1 -> Add/2
  Gain2/1 -> Derivative/1
  Derivative/1 -> Add/3

== system PID_sin_boques/PID/PD_psi ==
  errorpsi : Inport
  Add : Sum  Inputs=+++
  Derivative : Derivative
  Gain : Gain  Gain=Kp_psi
  Gain1 : Gain  Gain=1/Ti_psi
  Gain2 : Gain  Gain=Td_psi
  Integrator : Integrator
  U4 : Outport
  wires:
  errorpsi/1 -> Gain/1
  Add/1 -> U4/1
  Gain/1 -> Add/1, Gain1/1, Gain2/1
  Gain1/1 -> Integrator/1
  Integrator/1 -> Add/2
  Gain2/1 -> Derivative/1
  Derivative/1 -> Add/3

== system PID_sin_boques/PID/PD_theta ==
  errortheta : Inport
  Add : Sum  Inputs=+++
  Derivative : Derivative
  Gain : Gain  Gain=Kp_theta
  Gain1 : Gain  Gain=1/Ti_theta
  Gain2 : Gain  Gain=Td_theta
  Integrator : Integrator
  U3 : Outport
  wires:
  errortheta/1 -> Gain/1
  Add/1 -> U3/1
  Gain/1 -> Add/1, Gain1/1, Gain2/1
  Gain1/1 -> Integrator/1
  Integrator/1 -> Add/2
  Gain2/1 -> Derivative/1
  Derivative/1 -> Add/3

== system PID_sin_boques/PID/PD_z ==
  errorz : Inport
  Add : Sum  Inputs=+++
  Derivative : Derivative
  Gain : Gain  Gain=Kp_z
  Gain1 : Gain  Gain=1/Ti_z
  Gain2 : Gain  Gain=Td_z
  Integrator : Integrator
  U1 : Outport
  wires:
  errorz/1 -> Gain/1
  Add/1 -> U1/1
  Gain/1 -> Add/1, Gain1/1, Gain2/1
  Gain1/1 -> Integrator/1
  Integrator/1 -> Add/2
  Gain2/1 -> Derivative/1
  Derivative/1 -> Add/3

== system PID_sin_boques/QUADCOPTER/Angular body rates: p,q,r ==
  In1 : Inport
  Bus Creator : BusCreator  Inputs=3
  Bus Selector2 : BusSelector  OutputSignals=phi,theta,psi,phidot,thetadot,psidot
  Fcn : Fcn  Expr=u(4)-u(6)*sin(u(2))
  Fcn1 : Fcn  Expr=u(5)*cos(u(1))+u(6)*sin(u(1))*cos(u(2))
  Fcn2 : Fcn  Expr=-u(5)*sin(u(1))+u(6)*cos(u(1))*cos(u(2))
  Mux : Mux  Inputs=6
  Out1 : Outport
  wires:
  Bus Selector2/1 -> Mux/1  "<phi>"
  Bus Selector2/2 -> Mux/2  "<theta>"
  Bus Selector2/3 -> Mux/3  "<psi>"
  Bus Selector2/4 -> Mux/4  "<phidot>"
  Bus Selector2/5 -> Mux/5  "<thetadot>"
  Bus Selector2/6 -> Mux/6  "<psidot>"
  Mux/1 -> Fcn/1, Fcn2/1, Fcn1/1
  Fcn1/1 -> Bus Creator/2  "q"
  Fcn2/1 -> Bus Creator/3  "r"
  In1/1 -> Bus Selector2/1
  Bus Creator/1 -> Out1/1
  Fcn/1 -> Bus Creator/1  "p"

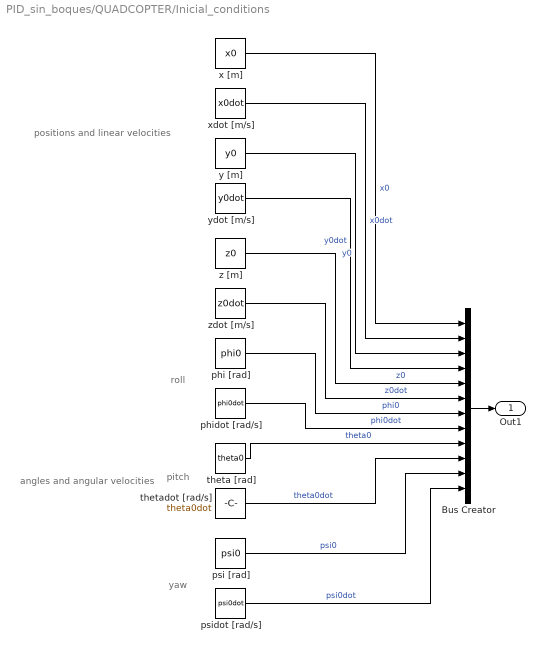
== system PID_sin_boques/QUADCOPTER/Inicial_conditions ==
  note: positions and linear velocities
  note: angles and angular velocities
  note: yaw
  note: pitch
  note: roll
  Bus Creator : BusCreator  Inputs=12
  phi [rad] : Constant  Value=phi0
  phidot [rad/s] : Constant  Value=phi0dot
  psi [rad] : Constant  Value=psi0
  psidot [rad/s] : Constant  Value=psi0dot
  theta [rad] : Constant  Value=theta0
  thetadot [rad/s] : Constant  Value=theta0dot
  x [m] : Constant  Value=x0
  xdot [m/s] : Constant  Value=x0dot
  y [m] : Constant  Value=y0
  ydot [m/s] : Constant  Value=y0dot
  z [m] : Constant  Value=z0
  zdot [m/s] : Constant  Value=z0dot
  Out1 : Outport
  wires:
  x [m]/1 -> Bus Creator/1  "x0"
  xdot [m/s]/1 -> Bus Creator/2  "x0dot"
  y [m]/1 -> Bus Creator/3  "y0"
  ydot [m/s]/1 -> Bus Creator/4  "y0dot"
  z [m]/1 -> Bus Creator/5  "z0"
  zdot [m/s]/1 -> Bus Creator/6  "z0dot"
  phi [rad]/1 -> Bus Creator/7  "phi0"
  phidot [rad/s]/1 -> Bus Creator/8  "phi0dot"
  theta [rad]/1 -> Bus Creator/9  "theta0"
  thetadot [rad/s]/1 -> Bus Creator/10  "theta0dot"
  psi [rad]/1 -> Bus Creator/11  "psi0"
  psidot [rad/s]/1 -> Bus Creator/12  "psi0dot"
  Bus Creator/1 -> Out1/1

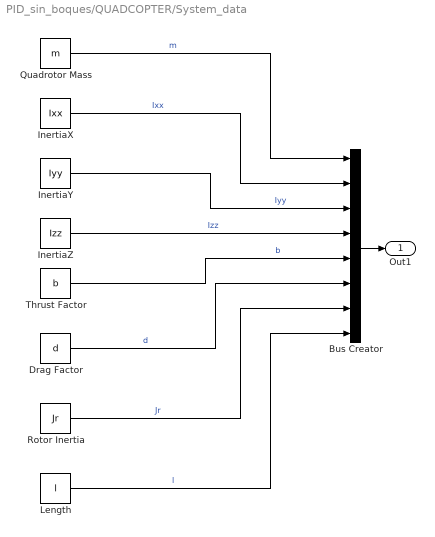
== system PID_sin_boques/QUADCOPTER/System_data ==
  Bus Creator : BusCreator  Inputs=8
  Drag Factor : Constant  Value=d
  InertiaX : Constant  Value=Ixx
  InertiaY : Constant  Value=Iyy
  InertiaZ : Constant  Value=Izz
  Length : Constant  Value=l
  Quadrotor Mass : Constant  Value=m
  Rotor Inertia : Constant  Value=Jr
  Thrust Factor : Constant  Value=b
  Out1 : Outport
  wires:
  Quadrotor Mass/1 -> Bus Creator/1  "m"
  InertiaX/1 -> Bus Creator/2  "Ixx"
  InertiaY/1 -> Bus Creator/3  "Iyy"
  InertiaZ/1 -> Bus Creator/4  "Izz"
  Thrust Factor/1 -> Bus Creator/5  "b"
  Drag Factor/1 -> Bus Creator/6  "d"
  Rotor Inertia/1 -> Bus Creator/7  "Jr"
  Length/1 -> Bus Creator/8  "l"
  Bus Creator/1 -> Out1/1

== system PID_sin_boques/QUADCOPTER/Velocity earth axis vX,vY,vZ ==
  In1 : Inport
  Bus Creator7 : BusCreator  Inputs=2
  Bus Selector3 : BusSelector  OutputSignals=xdot,ydot,zdot
  Fcn : Fcn  Expr=(u(1)^2+u(2)^2+u(3)^2)^(0.5)
  Mux : Mux  Inputs=3
  Out1 : Outport
  wires:
  Bus Selector3/1 -> Mux/1  "<xdot>"
  Bus Selector3/3 -> Mux/3  "<zdot>"
  Mux/1 -> Fcn/1, Bus Creator7/1
  Fcn/1 -> Bus Creator7/2  "v"
  In1/1 -> Bus Selector3/1
  Bus Creator7/1 -> Out1/1
  Bus Selector3/2 -> Mux/2  "<ydot>"

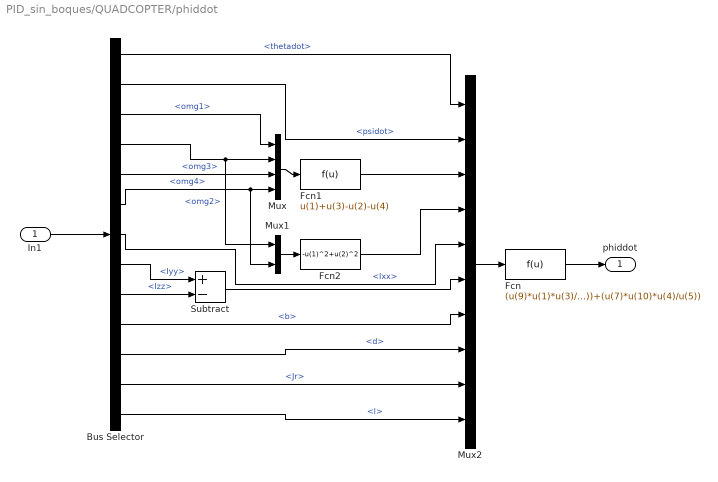
== system PID_sin_boques/QUADCOPTER/phiddot ==
  In1 : Inport
  Bus Selector : BusSelector  OutputSignals=States.thetadot,States.psidot,omg.omg1,omg.omg2,omg.omg3,omg.omg4,data.Ixx,data.Iyy,data.Izz,data.b,data.d,data.Jr,data.l
  Fcn : Fcn  Expr=(u(9)*u(1)*u(3)/u(5))+(u(6)*u(1)*u(2)/u(5))+(u(7)*u(10)*u(4)/u(5))
  Fcn1 : Fcn  Expr=u(1)+u(3)-u(2)-u(4)
  Fcn2 : Fcn  Expr=-u(1)^2+u(2)^2
  Mux : Mux
  Mux1 : Mux  Inputs=2
  Mux2 : Mux  Inputs=10
  Subtract : Sum  Inputs=+-
  phiddot : Outport
  wires:
  In1/1 -> Bus Selector/1
  Fcn/1 -> phiddot/1
  Mux/1 -> Fcn1/1
  Mux1/1 -> Fcn2/1
  Bus Selector/3 -> Mux/1  "<omg1>"
  Bus Selector/5 -> Mux/3  "<omg3>"
  Bus Selector/6 -> Mux/4, Mux1/2  "<omg4>"
  Bus Selector/8 -> Subtract/1  "<Iyy>"
  Bus Selector/9 -> Subtract/2  "<Izz>"
  Subtract/1 -> Mux2/6
  Mux2/1 -> Fcn/1
  Bus Selector/1 -> Mux2/1  "<thetadot>"
  Bus Selector/2 -> Mux2/2  "<psidot>"
  Fcn1/1 -> Mux2/3
  Fcn2/1 -> Mux2/4
  Bus Selector/7 -> Mux2/5  "<Ixx>"
  Bus Selector/10 -> Mux2/7  "<b>"
  Bus Selector/11 -> Mux2/8  "<d>"
  Bus Selector/12 -> Mux2/9  "<Jr>"
  Bus Selector/13 -> Mux2/10  "<l>"
  Bus Selector/4 -> Mux/2, Mux1/1  "<omg2>"

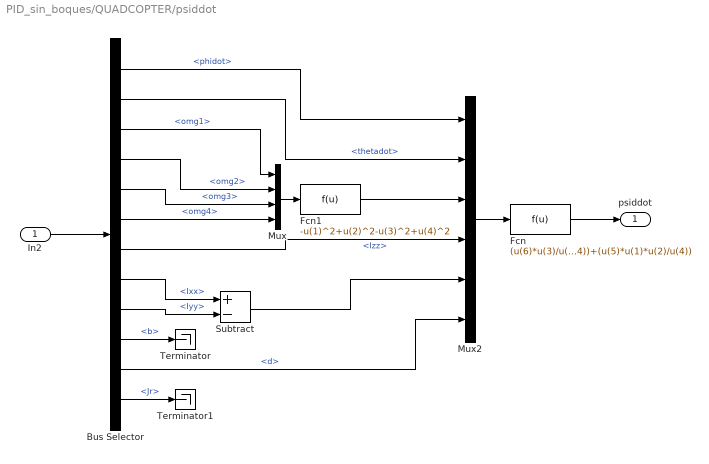
== system PID_sin_boques/QUADCOPTER/psiddot ==
  In2 : Inport
  Bus Selector : BusSelector  OutputSignals=States.phidot,States.thetadot,omg.omg1,omg.omg2,omg.omg3,omg.omg4,data.Izz,data.Ixx,data.Iyy,data.b,data.d,data.Jr
  Fcn : Fcn  Expr=(u(6)*u(3)/u(4))+(u(5)*u(1)*u(2)/u(4))
  Fcn1 : Fcn  Expr=-u(1)^2+u(2)^2-u(3)^2+u(4)^2
  Mux : Mux
  Mux2 : Mux  Inputs=6
  Subtract : Sum  Inputs=+-
  Terminator : Terminator
  Terminator1 : Terminator
  psiddot : Outport
  wires:
  In2/1 -> Bus Selector/1
  Fcn/1 -> psiddot/1
  Mux/1 -> Fcn1/1
  Bus Selector/3 -> Mux/1  "<omg1>"
  Bus Selector/4 -> Mux/2  "<omg2>"
  Bus Selector/5 -> Mux/3  "<omg3>"
  Bus Selector/6 -> Mux/4  "<omg4>"
  Mux2/1 -> Fcn/1
  Bus Selector/1 -> Mux2/1  "<phidot>"
  Fcn1/1 -> Mux2/3
  Bus Selector/2 -> Mux2/2  "<thetadot>"
  Bus Selector/8 -> Subtract/1  "<Ixx>"
  Bus Selector/9 -> Subtract/2  "<Iyy>"
  Bus Selector/10 -> Terminator/1  "<b>"
  Bus Selector/12 -> Terminator1/1  "<Jr>"
  Bus Selector/7 -> Mux2/4  "<Izz>"
  Subtract/1 -> Mux2/5
  Bus Selector/11 -> Mux2/6  "<d>"

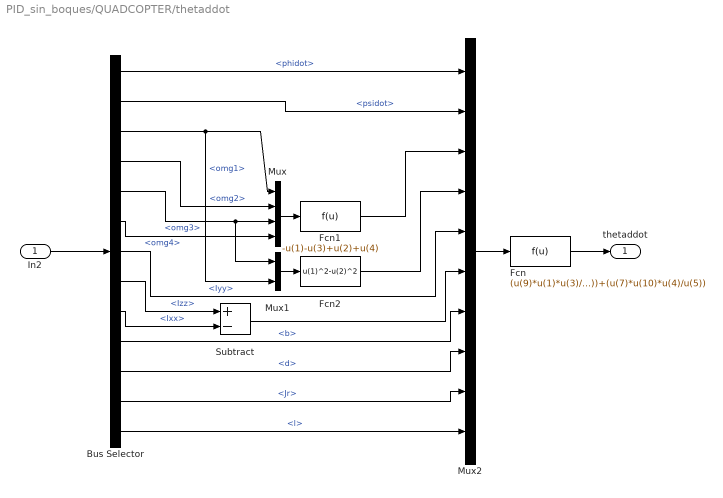
== system PID_sin_boques/QUADCOPTER/thetaddot ==
  In2 : Inport
  Bus Selector : BusSelector  OutputSignals=States.phidot,States.psidot,omg.omg1,omg.omg2,omg.omg3,omg.omg4,data.Iyy,data.Izz,data.Ixx,data.b,data.d,data.Jr,data.l
  Fcn : Fcn  Expr=(u(9)*u(1)*u(3)/u(5))+(u(6)*u(1)*u(2)/u(5))+(u(7)*u(10)*u(4)/u(5))
  Fcn1 : Fcn  Expr=-u(1)-u(3)+u(2)+u(4)
  Fcn2 : Fcn  Expr=u(1)^2-u(2)^2
  Mux : Mux
  Mux1 : Mux  Inputs=2
  Mux2 : Mux  Inputs=10
  Subtract : Sum  Inputs=+-
  thetaddot : Outport
  wires:
  In2/1 -> Bus Selector/1
  Fcn/1 -> thetaddot/1
  Mux/1 -> Fcn1/1
  Mux1/1 -> Fcn2/1
  Bus Selector/3 -> Mux/1, Mux1/2  "<omg1>"
  Bus Selector/4 -> Mux/2  "<omg2>"
  Bus Selector/5 -> Mux/3, Mux1/1  "<omg3>"
  Bus Selector/6 -> Mux/4  "<omg4>"
  Bus Selector/7 -> Mux2/5  "<Iyy>"
  Bus Selector/8 -> Subtract/1  "<Izz>"
  Mux2/1 -> Fcn/1
  Bus Selector/1 -> Mux2/1  "<phidot>"
  Bus Selector/2 -> Mux2/2  "<psidot>"
  Fcn1/1 -> Mux2/3
  Fcn2/1 -> Mux2/4
  Bus Selector/10 -> Mux2/7  "<b>"
  Bus Selector/11 -> Mux2/8  "<d>"
  Bus Selector/12 -> Mux2/9  "<Jr>"
  Bus Selector/9 -> Subtract/2  "<Ixx>"
  Subtract/1 -> Mux2/6
  Bus Selector/13 -> Mux2/10  "<l>"

== system PID_sin_boques/QUADCOPTER/xddot ==
  In1 : Inport
  Bus Selector : BusSelector  OutputSignals=data.m,data.b,omg.omg1,omg.omg2,omg.omg3,omg.omg4,States.phi,States.theta,States.psi
  Fcn : Fcn  Expr=u(2)*(u(3)^2+u(4)^2+u(5)^2+u(6)^2)/u(1)
  Fcn1 : Fcn  Expr=u(1)*(cos(u(2))*sin(u(3))*cos(u(4))+sin(u(2))*sin(u(4)))
  Mux : Mux  Inputs=6
  Mux3 : Mux
  Out1 : Outport
  wires:
  In1/1 -> Bus Selector/1
  Bus Selector/1 -> Mux/1  "<m>"
  Bus Selector/2 -> Mux/2  "<b>"
  Bus Selector/3 -> Mux/3  "<omg1>"
  Bus Selector/4 -> Mux/4  "<omg2>"
  Bus Selector/5 -> Mux/5  "<omg3>"
  Bus Selector/6 -> Mux/6  "<omg4>"
  Mux/1 -> Fcn/1
  Bus Selector/7 -> Mux3/2  "<phi>"
  Bus Selector/8 -> Mux3/3  "<theta>"
  Bus Selector/9 -> Mux3/4  "<psi>"
  Fcn1/1 -> Out1/1
  Mux3/1 -> Fcn1/1
  Fcn/1 -> Mux3/1

== system PID_sin_boques/QUADCOPTER/yddot ==
  In1 : Inport
  Bus Selector : BusSelector  OutputSignals=data.m,data.b,omg.omg1,omg.omg2,omg.omg3,omg.omg4,States.phi,States.theta,States.psi
  Fcn : Fcn  Expr=u(2)*(u(3)^2+u(4)^2+u(5)^2+u(6)^2)/u(1)
  Fcn1 : Fcn  Expr=u(1)*(cos(u(2))*sin(u(3))*sin(u(4))-sin(u(2))*cos(u(4)))
  Mux : Mux  Inputs=6
  Mux3 : Mux
  Out1 : Outport
  wires:
  In1/1 -> Bus Selector/1
  Bus Selector/1 -> Mux/1  "<m>"
  Bus Selector/2 -> Mux/2  "<b>"
  Bus Selector/3 -> Mux/3  "<omg1>"
  Bus Selector/4 -> Mux/4  "<omg2>"
  Bus Selector/5 -> Mux/5  "<omg3>"
  Bus Selector/6 -> Mux/6  "<omg4>"
  Mux/1 -> Fcn/1
  Bus Selector/9 -> Mux3/4  "<psi>"
  Fcn1/1 -> Out1/1
  Mux3/1 -> Fcn1/1
  Fcn/1 -> Mux3/1
  Bus Selector/7 -> Mux3/2  "<phi>"
  Bus Selector/8 -> Mux3/3  "<theta>"

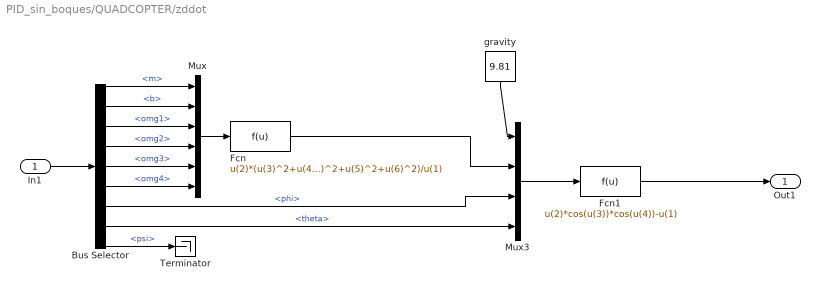
== system PID_sin_boques/QUADCOPTER/zddot ==
  In1 : Inport
  Bus Selector : BusSelector  OutputSignals=data.m,data.b,omg.omg1,omg.omg2,omg.omg3,omg.omg4,States.phi,States.theta,States.psi
  Fcn : Fcn  Expr=u(2)*(u(3)^2+u(4)^2+u(5)^2+u(6)^2)/u(1)
  Fcn1 : Fcn  Expr=u(2)*cos(u(3))*cos(u(4))-u(1)
  Mux : Mux  Inputs=6
  Mux3 : Mux
  Terminator : Terminator
  gravity : Constant  Value=9.81
  Out1 : Outport
  wires:
  In1/1 -> Bus Selector/1
  Bus Selector/1 -> Mux/1  "<m>"
  Bus Selector/2 -> Mux/2  "<b>"
  Bus Selector/3 -> Mux/3  "<omg1>"
  Bus Selector/4 -> Mux/4  "<omg2>"
  Bus Selector/5 -> Mux/5  "<omg3>"
  Bus Selector/6 -> Mux/6  "<omg4>"
  Mux/1 -> Fcn/1
  Fcn1/1 -> Out1/1
  Mux3/1 -> Fcn1/1
  gravity/1 -> Mux3/1
  Fcn/1 -> Mux3/2
  Bus Selector/9 -> Terminator/1  "<psi>"
  Bus Selector/7 -> Mux3/3  "<phi>"
  Bus Selector/8 -> Mux3/4  "<theta>"
